simulink library "intraSpoolingController_ul"  (R2018b)
settings: Solver=VariableStepAuto  StartTime=0.0  StopTime=10.0  RelTol=1e-3
undefined symbols (not defined in the file or in its folder): pathCtrl
libraries: firstOrderFilter_ul x1
settings Model: Creator=James Reed  LastModifiedBy=jldanie5

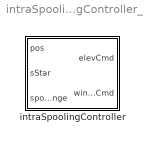
== system intraSpoolingController_ul ==
  intraSpoolingController : Subsystem

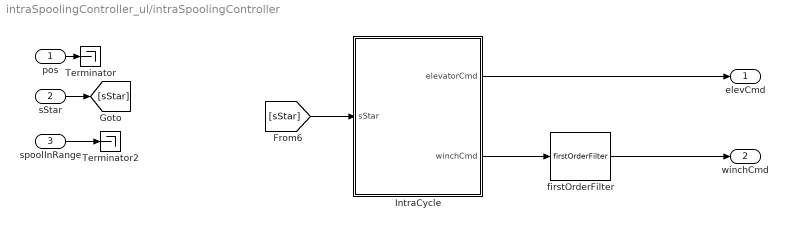
== system intraSpoolingController_ul/intraSpoolingController ==
  pos : Inport
  "sStar " : Inport  Port=2
  spoolInRange : Inport  Port=3
  IntraCycle : Stateflow chart  TreatAsAtomicUnit=on  mask{reelInSpd=pathCtrl.winchSpeedIn.Value, reelOutSpd=pathCtrl.winchSpeedOut.Value, ranges=pathCtrl.outRanges.Value, elevatorReelInDef=pathCtrl.elevatorReelInDef.Value}
      mask prompts: reelInSpd "Spool in speed"; reelOutSpd "Spool out speed"; ranges "Ranges to spool out"; elevatorReelInDef "Elevator Defection during Spool In"
  Terminator : Terminator
  Terminator2 : Terminator
  firstOrderFilter : firstOrderFilter_ul/firstOrderFilter  tau=1  ic=0
  elevCmd : Outport
  "winchCmd " : Outport  Port=2
  wires:
  firstOrderFilter/1 -> "winchCmd "/1
  [sStar] -> IntraCycle/1(sStar)
  IntraCycle/1(elevatorCmd) -> elevCmd/1
  IntraCycle/2(winchCmd) -> firstOrderFilter/1
  "sStar "/1 -> [sStar]
  pos/1 -> Terminator/1
  spoolInRange/1 -> Terminator2/1

== stateflow chart intraSpoolingController_ul/intraSpoolingController/IntraCycle ==
  state ReelIn
    entry:
    elevatorCmd= elevatorReelInDef;
    winchCmd = reelInSpd;
  state ReelOut
    entry:
    winchCmd = reelOutSpd;
    elevatorCmd= 0;
  (default) -> ReelOut
  ReelOut -> ReelIn : [ ~any(and(sStar>=ranges(:,1),sStar<ranges(:,2)))]
  ReelIn -> ReelOut : [any(and(sStar>=ranges(:,1),sStar<ranges(:,2)))]
  data: elevatorCmd output; sStar input; winchCmd output; elevatorReelInDef parameter; reelInSpd parameter; reelOutSpd parameter; ranges parameter
